simulink model "pd_path_sg"  (R2013b)
settings: Solver=ode45  StartTime=0.0  StopTime=10  RelTol=1e-3
undefined symbols (not defined in the file or in its folder): A, A2, B, C, D, EVAL, i, output_samp_bcoef, PCIN, reg_pk_lim, reg_plim, reg_scale, reg_sr_lim, reg_staclr, reg_txgain, THIS_DATE, W, X, Z
undefined symbols (not defined in the file): lut_address, lut_address_s5, reg_dltap
libraries: xbsIndex_r4 x3819, lut_ram_vhdl x32
(part 1 of 31)
settings Model: Creator=eyonfen  LastModifiedBy=Administrator
settings DataIOCC: SignalLoggingSaveFormat=ModelDataLogs
settings OptimizationCC: ExpressionDepthLimit=2147483647
settings DebuggingCC: FcnCallInpInsideContextMsg=EnableAllAsWarning  FrameProcessingCompatibilityMsg=error  StateNameClashWarn=warning
settings GRTTargetCC: CodeReplacementLibrary=None  CPPClassGenCompliant=on

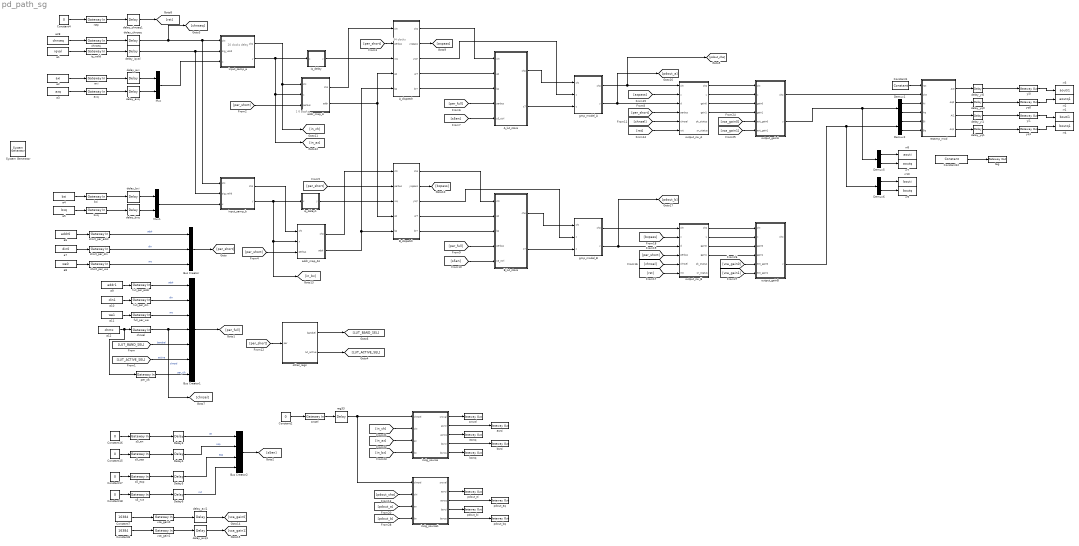
== system pd_path_sg ==
  note: 1 6 clocks
  note: 20 clocks delay
  note: 34 clocks
  " System Generator" : xbsIndex_r4/ System Generator  Tag=genX  xilinxfamily=zynquplus  part=xczu15eg  speed=-1LV-i-EVAL  package=ffvb1156  synthesis_tool=Vivado  clock_wrapper=Clock Enables  directory=../../../netlist/pd_path_sg  proj_type=Vivado  Synth_file=Vivado Synthesis Defaults  Impl_file=Vivado Implementation Defaults  testbench=off  simulink_period=1  sysclk_period=10  dcm_input_clock_period=10  incr_netlist=off  trim_vbits=Everywhere in SubSystem  dbl_ovrd=According to Block Masks  core_generation=According to Block Masks  run_coregen=off  deprecated_control=off  eval_field=0  block_type=sysgen
  A_dispatch : Subsystem  mask{para_band=0}
  A_lut_store : Subsystem  mask{band_sel=0}
  B_dispatch : Subsystem  mask{para_band=1}
  B_lut_store : Subsystem  mask{band_sel=1}
  Bus Creator : BusCreator  Inputs=3
  Bus Creator1 : BusCreator  Inputs=7
  Bus Creator2 : BusCreator
  Constant1 : xbsIndex_r4/Constant  const=0  gui_display_data_type=Boolean  arith_type=Boolean  n_bits=10  bin_pt=0  preci_type=Single  exp_width=8  frac_width=24  explicit_period=on  period=1  equ=P=C  opselect=C  inp2=PCIN>>17  opr=+  inp1=P  carry=CIN  dbl_ovrd=off  block_type=constant
  Constant12 : xbsIndex_r4/Constant  const=THIS_DATE  gui_display_data_type=Fixed-point  arith_type=Unsigned  n_bits=32  bin_pt=0  preci_type=Single  exp_width=8  frac_width=24  explicit_period=off  period=1  equ=P=C  opselect=C  inp2=PCIN>>17  opr=+  inp1=P  carry=CIN  dbl_ovrd=off  block_type=constant
  Constant{2,4,15..18} (6 alike) : Constant  Value=0
  Constant7 : Constant  Value=16384
  Constant8 : Constant  Value=16384
  Delay{3..6} (4 alike) : xbsIndex_r4/Delay  rst=off  infoeditControl=Selection of Reset will increase slice count due to use of real FFs and instead of SRLs  en=off  latency=1  reg_retiming=off  dbl_ovrd=off  block_type=delay
  Demux{1..2,5..6} (4 alike) : Demux  Outputs=2
  Mux : Mux  Inputs=2
  Mux1 : Mux  Inputs=2
  a1 : FromWorkspace  VariableName=iqval  Interpolate=off  OutputAfterFinalValue=Cyclic repetition
  a10 : FromWorkspace  VariableName=din1  Interpolate=off  OutputAfterFinalValue=Setting to zero
  a11 : FromWorkspace  VariableName=we1  Interpolate=off  OutputAfterFinalValue=Setting to zero
  a12 : FromWorkspace  VariableName=chntx  Interpolate=off  OutputAfterFinalValue=Cyclic repetition
  a2 : FromWorkspace  VariableName=axi  Interpolate=off  OutputAfterFinalValue=Setting to zero
  a28 : FromWorkspace  VariableName=chnseq  Interpolate=off  OutputAfterFinalValue=Cyclic repetition
  a3 : FromWorkspace  VariableName=axq  Interpolate=off  OutputAfterFinalValue=Setting to zero
  a4 : FromWorkspace  VariableName=bxi  Interpolate=off  OutputAfterFinalValue=Setting to zero
  a5 : FromWorkspace  VariableName=bxq  Interpolate=off  OutputAfterFinalValue=Setting to zero
  a6 : FromWorkspace  VariableName=addr0  Interpolate=off  OutputAfterFinalValue=Setting to zero
  a7 : FromWorkspace  VariableName=din0  Interpolate=off  OutputAfterFinalValue=Setting to zero
  a8 : FromWorkspace  VariableName=we0  Interpolate=off  OutputAfterFinalValue=Setting to zero
  a9 : FromWorkspace  VariableName=addr1  Interpolate=off  OutputAfterFinalValue=Setting to zero
  addr_map_A : Subsystem  mask{para_band=0}
  addr_map_A1 : Subsystem  mask{para_band=1}
  asrci : xbsIndex_r4/Gateway Out  inherit_from_input=off  hdl_port=on  rows=1  columns=1  UseAsDAC=off  DACChannel='1'  interface=None  automatic_assignment=on  address_offset=hex2dec('00')  intf_name=''  intf_description=''  timing_constraint=None  locs_specified=off  LOCs={}  io_standard={}  block_type=gatewayout
  asrcq : xbsIndex_r4/Gateway Out  inherit_from_input=off  hdl_port=on  rows=1  columns=1  UseAsDAC=off  DACChannel='1'  interface=None  automatic_assignment=on  address_offset=hex2dec('00')  intf_name=''  intf_description=''  timing_constraint=None  locs_specified=off  LOCs={}  io_standard={}  block_type=gatewayout
  axi : xbsIndex_r4/Gateway In  gui_display_data_type=Fixed-point  arith_type="Signed  (2's comp)"  n_bits=16  bin_pt=0  preci_type=Single  exp_width=8  frac_width=24  rows=1  columns=1  quantization="Round  (unbiased: +/- Inf)"  overflow=Saturate  period=1  UseAsADC=off  ADCChannel='1'  interface=None  automatic_assignment=on  address_offset=hex2dec('00')  intf_name=''  intf_description=''  default_value=0  timing_constraint=None  locs_specified=off  LOCs={}  io_standard={}  inherit_from_input=off  hdl_port=on  dbl_ovrd=off  block_type=gatewayin
  axq : xbsIndex_r4/Gateway In  gui_display_data_type=Fixed-point  arith_type="Signed  (2's comp)"  n_bits=16  bin_pt=0  preci_type=Single  exp_width=8  frac_width=24  rows=1  columns=1  quantization="Round  (unbiased: +/- Inf)"  overflow=Saturate  period=1  UseAsADC=off  ADCChannel='1'  interface=None  automatic_assignment=on  address_offset=hex2dec('00')  intf_name=''  intf_description=''  default_value=0  timing_constraint=None  locs_specified=off  LOCs={}  io_standard={}  inherit_from_input=off  hdl_port=on  dbl_ovrd=off  block_type=gatewayin
  bsrci : xbsIndex_r4/Gateway Out  inherit_from_input=off  hdl_port=on  rows=1  columns=1  UseAsDAC=off  DACChannel='1'  interface=None  automatic_assignment=on  address_offset=hex2dec('00')  intf_name=''  intf_description=''  timing_constraint=None  locs_specified=off  LOCs={}  io_standard={}  block_type=gatewayout
  bsrcq : xbsIndex_r4/Gateway Out  inherit_from_input=off  hdl_port=on  rows=1  columns=1  UseAsDAC=off  DACChannel='1'  interface=None  automatic_assignment=on  address_offset=hex2dec('00')  intf_name=''  intf_description=''  timing_constraint=None  locs_specified=off  LOCs={}  io_standard={}  block_type=gatewayout
  bxi : xbsIndex_r4/Gateway In  gui_display_data_type=Fixed-point  arith_type="Signed  (2's comp)"  n_bits=16  bin_pt=0  preci_type=Single  exp_width=8  frac_width=24  rows=1  columns=1  quantization="Round  (unbiased: +/- Inf)"  overflow=Saturate  period=1  UseAsADC=off  ADCChannel='1'  interface=None  automatic_assignment=on  address_offset=hex2dec('00')  intf_name=''  intf_description=''  default_value=0  timing_constraint=None  locs_specified=off  LOCs={}  io_standard={}  inherit_from_input=off  hdl_port=on  dbl_ovrd=off  block_type=gatewayin
  bxq : xbsIndex_r4/Gateway In  gui_display_data_type=Fixed-point  arith_type="Signed  (2's comp)"  n_bits=16  bin_pt=0  preci_type=Single  exp_width=8  frac_width=24  rows=1  columns=1  quantization="Round  (unbiased: +/- Inf)"  overflow=Saturate  period=1  UseAsADC=off  ADCChannel='1'  interface=None  automatic_assignment=on  address_offset=hex2dec('00')  intf_name=''  intf_description=''  default_value=0  timing_constraint=None  locs_specified=off  LOCs={}  io_standard={}  inherit_from_input=off  hdl_port=on  dbl_ovrd=off  block_type=gatewayin
  chnsel : xbsIndex_r4/Gateway In  gui_display_data_type=Fixed-point  arith_type=Unsigned  n_bits=1  bin_pt=0  preci_type=Single  exp_width=8  frac_width=24  rows=1  columns=1  quantization="Round  (unbiased: +/- Inf)"  overflow=Saturate  period=1  UseAsADC=off  ADCChannel='1'  interface=None  automatic_assignment=on  address_offset=hex2dec('00')  intf_name=''  intf_description=''  default_value=0  timing_constraint=None  locs_specified=off  LOCs={}  io_standard={}  inherit_from_input=off  hdl_port=on  dbl_ovrd=off  block_type=gatewayin
  chnseq : xbsIndex_r4/Gateway In  gui_display_data_type=Fixed-point  arith_type=Unsigned  n_bits=1  bin_pt=0  preci_type=Single  exp_width=8  frac_width=24  rows=1  columns=1  quantization="Round  (unbiased: +/- Inf)"  overflow=Saturate  period=1  UseAsADC=off  ADCChannel='1'  interface=None  automatic_assignment=on  address_offset=hex2dec('00')  intf_name=''  intf_description=''  default_value=0  timing_constraint=None  locs_specified=off  LOCs={}  io_standard={}  inherit_from_input=off  hdl_port=on  dbl_ovrd=off  block_type=gatewayin
  delay_axi : xbsIndex_r4/Delay  rst=off  infoeditControl=Selection of Reset will increase slice count due to use of real FFs and instead of SRLs  en=off  latency=1  reg_retiming=off  dbl_ovrd=off  block_type=delay
  delay_axi1 : xbsIndex_r4/Delay  rst=off  infoeditControl=Selection of Reset will increase slice count due to use of real FFs and instead of SRLs  en=off  latency=1  reg_retiming=off  dbl_ovrd=off  block_type=delay
  delay_axq : xbsIndex_r4/Delay  rst=off  infoeditControl=Selection of Reset will increase slice count due to use of real FFs and instead of SRLs  en=off  latency=1  reg_retiming=off  dbl_ovrd=off  block_type=delay
  delay_axq1 : xbsIndex_r4/Delay  rst=off  infoeditControl=Selection of Reset will increase slice count due to use of real FFs and instead of SRLs  en=off  latency=1  reg_retiming=off  dbl_ovrd=off  block_type=delay
  delay_bxi : xbsIndex_r4/Delay  rst=off  infoeditControl=Selection of Reset will increase slice count due to use of real FFs and instead of SRLs  en=off  latency=1  reg_retiming=off  dbl_ovrd=off  block_type=delay
  delay_bxq : xbsIndex_r4/Delay  rst=off  infoeditControl=Selection of Reset will increase slice count due to use of real FFs and instead of SRLs  en=off  latency=1  reg_retiming=off  dbl_ovrd=off  block_type=delay
  delay_chnseq : xbsIndex_r4/Delay  rst=off  infoeditControl=Selection of Reset will increase slice count due to use of real FFs and instead of SRLs  en=off  latency=1  reg_retiming=off  dbl_ovrd=off  block_type=delay
  delay_chnseq1 : xbsIndex_r4/Delay  rst=off  infoeditControl=Selection of Reset will increase slice count due to use of real FFs and instead of SRLs  en=off  latency=2  reg_retiming=off  dbl_ovrd=off  block_type=delay
      settings: infoedit=Hardware notes: A delay line is a chain, each link of which is an SRL16 or SRL32 followed by a flip-flop.
  delay_iqval : xbsIndex_r4/Delay  rst=off  infoeditControl=Selection of Reset will increase slice count due to use of real FFs and instead of SRLs  en=off  latency=1  reg_retiming=off  dbl_ovrd=off  block_type=delay
  delay_yi0 : xbsIndex_r4/Delay  rst=off  infoeditControl=Selection of Reset will increase slice count due to use of real FFs and instead of SRLs  en=off  latency=1  reg_retiming=off  dbl_ovrd=off  block_type=delay
  delay_yi1 : xbsIndex_r4/Delay  rst=off  infoeditControl=Selection of Reset will increase slice count due to use of real FFs and instead of SRLs  en=off  latency=1  reg_retiming=off  dbl_ovrd=off  block_type=delay
  delay_yq0 : xbsIndex_r4/Delay  rst=off  infoeditControl=Selection of Reset will increase slice count due to use of real FFs and instead of SRLs  en=off  latency=1  reg_retiming=off  dbl_ovrd=off  block_type=delay
  delay_yq1 : xbsIndex_r4/Delay  rst=off  infoeditControl=Selection of Reset will increase slice count due to use of real FFs and instead of SRLs  en=off  latency=1  reg_retiming=off  dbl_ovrd=off  block_type=delay
  full_per_addr : xbsIndex_r4/Gateway In  gui_display_data_type=Fixed-point  arith_type=Unsigned  n_bits=20  bin_pt=0  preci_type=Single  exp_width=8  frac_width=24  rows=1  columns=1  quantization="Round  (unbiased: +/- Inf)"  overflow=Saturate  period=1  UseAsADC=off  ADCChannel='1'  interface=None  automatic_assignment=on  address_offset=hex2dec('00')  intf_name=''  intf_description=''  default_value=0  timing_constraint=None  locs_specified=off  LOCs={}  io_standard={}  inherit_from_input=off  hdl_port=on  dbl_ovrd=off  block_type=gatewayin
  full_per_din : xbsIndex_r4/Gateway In  gui_display_data_type=Fixed-point  arith_type=Unsigned  n_bits=32  bin_pt=0  preci_type=Single  exp_width=8  frac_width=24  rows=1  columns=1  quantization="Round  (unbiased: +/- Inf)"  overflow=Saturate  period=1  UseAsADC=off  ADCChannel='1'  interface=None  automatic_assignment=on  address_offset=hex2dec('00')  intf_name=''  intf_description=''  default_value=0  timing_constraint=None  locs_specified=off  LOCs={}  io_standard={}  inherit_from_input=off  hdl_port=on  dbl_ovrd=off  block_type=gatewayin
  full_per_we : xbsIndex_r4/Gateway In  gui_display_data_type=Boolean  arith_type=Boolean  n_bits=1  bin_pt=0  preci_type=Single  exp_width=8  frac_width=24  rows=1  columns=1  quantization="Round  (unbiased: +/- Inf)"  overflow=Saturate  period=1  UseAsADC=off  ADCChannel='1'  interface=None  automatic_assignment=on  address_offset=hex2dec('00')  intf_name=''  intf_description=''  default_value=0  timing_constraint=None  locs_specified=off  LOCs={}  io_standard={}  inherit_from_input=off  hdl_port=on  dbl_ovrd=off  block_type=gatewayin
  gmp_model_A : Subsystem
  gmp_model_B : Subsystem
  input_samp_a : Subsystem
  input_samp_b : Subsystem
  insig_source : Subsystem
  insig_source1 : Subsystem
  iq_delay : Subsystem  mask{clocks=30}
  iq_delay1 : Subsystem  mask{clocks=30}
  iq_valid : xbsIndex_r4/Gateway In  gui_display_data_type=Fixed-point  arith_type=Unsigned  n_bits=1  bin_pt=0  preci_type=Single  exp_width=8  frac_width=24  rows=1  columns=1  quantization="Round  (unbiased: +/- Inf)"  overflow=Saturate  period=1  UseAsADC=off  ADCChannel='1'  interface=None  automatic_assignment=on  address_offset=hex2dec('00')  intf_name=''  intf_description=''  default_value=0  timing_constraint=None  locs_specified=off  LOCs={}  io_standard={}  inherit_from_input=off  hdl_port=on  dbl_ovrd=off  block_type=gatewayin
  other_regs : Subsystem
  output_gainA : Subsystem
  output_gainB : Subsystem
  output_sw_A : Subsystem  mask{para_band=0}
  output_sw_B : Subsystem  mask{para_band=1}
  pdout_ai : xbsIndex_r4/Gateway Out  inherit_from_input=off  hdl_port=on  rows=1  columns=1  UseAsDAC=off  DACChannel='1'  interface=None  automatic_assignment=on  address_offset=hex2dec('00')  intf_name=''  intf_description=''  timing_constraint=None  locs_specified=off  LOCs={}  io_standard={}  block_type=gatewayout
  pdout_aq : xbsIndex_r4/Gateway Out  inherit_from_input=off  hdl_port=on  rows=1  columns=1  UseAsDAC=off  DACChannel='1'  interface=None  automatic_assignment=on  address_offset=hex2dec('00')  intf_name=''  intf_description=''  timing_constraint=None  locs_specified=off  LOCs={}  io_standard={}  block_type=gatewayout
  pdout_bi : xbsIndex_r4/Gateway Out  inherit_from_input=off  hdl_port=on  rows=1  columns=1  UseAsDAC=off  DACChannel='1'  interface=None  automatic_assignment=on  address_offset=hex2dec('00')  intf_name=''  intf_description=''  timing_constraint=None  locs_specified=off  LOCs={}  io_standard={}  block_type=gatewayout
  pdout_bq : xbsIndex_r4/Gateway Out  inherit_from_input=off  hdl_port=on  rows=1  columns=1  UseAsDAC=off  DACChannel='1'  interface=None  automatic_assignment=on  address_offset=hex2dec('00')  intf_name=''  intf_description=''  timing_constraint=None  locs_specified=off  LOCs={}  io_standard={}  block_type=gatewayout
  per_clk : xbsIndex_r4/Gateway In  gui_display_data_type=Fixed-point  arith_type=Unsigned  n_bits=1  bin_pt=0  preci_type=Single  exp_width=8  frac_width=24  rows=1  columns=1  quantization="Round  (unbiased: +/- Inf)"  overflow=Saturate  period=1  UseAsADC=off  ADCChannel='1'  interface=None  automatic_assignment=on  address_offset=hex2dec('00')  intf_name=''  intf_description=''  default_value=0  timing_constraint=None  locs_specified=off  LOCs={}  io_standard={}  inherit_from_input=off  hdl_port=on  dbl_ovrd=off  block_type=gatewayin
  reg33 : xbsIndex_r4/Delay  rst=off  infoeditControl=Selection of Reset will increase slice count due to use of real FFs and instead of SRLs  en=off  latency=1  reg_retiming=off  dbl_ovrd=off  block_type=delay
  resamp_mod : Subsystem
  rr1 : ToWorkspace  VariableName=bouti1  SampleTime=-1
  rr10 : ToWorkspace  VariableName=bouti  SampleTime=-1
  rr2 : ToWorkspace  VariableName=aoutq1  SampleTime=-1
  rr3 : ToWorkspace  VariableName=aouti1  SampleTime=-1
  rr4 : ToWorkspace  VariableName=boutq1  SampleTime=-1
  rr7 : ToWorkspace  VariableName=aoutq  SampleTime=-1
  rr8 : ToWorkspace  VariableName=aouti  SampleTime=-1
  rr9 : ToWorkspace  VariableName=boutq  SampleTime=-1
  rstp : xbsIndex_r4/Gateway In  gui_display_data_type=Boolean  arith_type=Boolean  n_bits=1  bin_pt=0  preci_type=Single  exp_width=8  frac_width=24  rows=1  columns=1  quantization="Round  (unbiased: +/- Inf)"  overflow=Saturate  period=1  UseAsADC=off  ADCChannel='1'  interface=None  automatic_assignment=on  address_offset=hex2dec('00')  intf_name=''  intf_description=''  default_value=0  timing_constraint=None  locs_specified=off  LOCs={}  io_standard={}  inherit_from_input=off  hdl_port=on  dbl_ovrd=off  block_type=gatewayin
  s5_en : xbsIndex_r4/Gateway In  gui_display_data_type=Boolean  arith_type=Boolean  n_bits=1  bin_pt=0  preci_type=Single  exp_width=8  frac_width=24  rows=1  columns=1  quantization="Round  (unbiased: +/- Inf)"  overflow=Saturate  period=1  UseAsADC=off  ADCChannel='1'  interface=None  automatic_assignment=on  address_offset=hex2dec('00')  intf_name=''  intf_description=''  default_value=0  timing_constraint=None  locs_specified=off  LOCs={}  io_standard={}  inherit_from_input=off  hdl_port=on  dbl_ovrd=off  block_type=gatewayin
  s5_eop : xbsIndex_r4/Gateway In  gui_display_data_type=Boolean  arith_type=Boolean  n_bits=1  bin_pt=0  preci_type=Single  exp_width=8  frac_width=24  rows=1  columns=1  quantization="Round  (unbiased: +/- Inf)"  overflow=Saturate  period=1  UseAsADC=off  ADCChannel='1'  interface=None  automatic_assignment=on  address_offset=hex2dec('00')  intf_name=''  intf_description=''  default_value=0  timing_constraint=None  locs_specified=off  LOCs={}  io_standard={}  inherit_from_input=off  hdl_port=on  dbl_ovrd=off  block_type=gatewayin
  s5_nxt : xbsIndex_r4/Gateway In  gui_display_data_type=Boolean  arith_type=Boolean  n_bits=1  bin_pt=0  preci_type=Single  exp_width=8  frac_width=24  rows=1  columns=1  quantization="Round  (unbiased: +/- Inf)"  overflow=Saturate  period=1  UseAsADC=off  ADCChannel='1'  interface=None  automatic_assignment=on  address_offset=hex2dec('00')  intf_name=''  intf_description=''  default_value=0  timing_constraint=None  locs_specified=off  LOCs={}  io_standard={}  inherit_from_input=off  hdl_port=on  dbl_ovrd=off  block_type=gatewayin
  s5_sop : xbsIndex_r4/Gateway In  gui_display_data_type=Boolean  arith_type=Boolean  n_bits=1  bin_pt=0  preci_type=Single  exp_width=8  frac_width=24  rows=1  columns=1  quantization="Round  (unbiased: +/- Inf)"  overflow=Saturate  period=1  UseAsADC=off  ADCChannel='1'  interface=None  automatic_assignment=on  address_offset=hex2dec('00')  intf_name=''  intf_description=''  default_value=0  timing_constraint=None  locs_specified=off  LOCs={}  io_standard={}  inherit_from_input=off  hdl_port=on  dbl_ovrd=off  block_type=gatewayin
  short_per_addr : xbsIndex_r4/Gateway In  gui_display_data_type=Fixed-point  arith_type=Unsigned  n_bits=12  bin_pt=0  preci_type=Single  exp_width=8  frac_width=24  rows=1  columns=1  quantization="Round  (unbiased: +/- Inf)"  overflow=Saturate  period=1  UseAsADC=off  ADCChannel='1'  interface=None  automatic_assignment=on  address_offset=hex2dec('00')  intf_name=''  intf_description=''  default_value=0  timing_constraint=None  locs_specified=off  LOCs={}  io_standard={}  inherit_from_input=off  hdl_port=on  dbl_ovrd=off  block_type=gatewayin
  short_per_din : xbsIndex_r4/Gateway In  gui_display_data_type=Fixed-point  arith_type=Unsigned  n_bits=32  bin_pt=0  preci_type=Single  exp_width=8  frac_width=24  rows=1  columns=1  quantization="Round  (unbiased: +/- Inf)"  overflow=Saturate  period=1  UseAsADC=off  ADCChannel='1'  interface=None  automatic_assignment=on  address_offset=hex2dec('00')  intf_name=''  intf_description=''  default_value=0  timing_constraint=None  locs_specified=off  LOCs={}  io_standard={}  inherit_from_input=off  hdl_port=on  dbl_ovrd=off  block_type=gatewayin
  short_per_we : xbsIndex_r4/Gateway In  gui_display_data_type=Boolean  arith_type=Boolean  n_bits=1  bin_pt=0  preci_type=Single  exp_width=8  frac_width=24  rows=1  columns=1  quantization="Round  (unbiased: +/- Inf)"  overflow=Saturate  period=1  UseAsADC=off  ADCChannel='1'  interface=None  automatic_assignment=on  address_offset=hex2dec('00')  intf_name=''  intf_description=''  default_value=0  timing_constraint=None  locs_specified=off  LOCs={}  io_standard={}  inherit_from_input=off  hdl_port=on  dbl_ovrd=off  block_type=gatewayin
  srcsel : xbsIndex_r4/Gateway In  gui_display_data_type=Fixed-point  arith_type=Unsigned  n_bits=1  bin_pt=0  preci_type=Single  exp_width=8  frac_width=24  rows=1  columns=1  quantization="Round  (unbiased: +/- Inf)"  overflow=Saturate  period=1  UseAsADC=off  ADCChannel='1'  interface=None  automatic_assignment=on  address_offset=hex2dec('00')  intf_name=''  intf_description=''  default_value=0  timing_constraint=None  locs_specified=off  LOCs={}  io_standard={}  inherit_from_input=off  hdl_port=on  dbl_ovrd=off  block_type=gatewayin
  srcval : xbsIndex_r4/Gateway Out  inherit_from_input=off  hdl_port=on  rows=1  columns=1  UseAsDAC=off  DACChannel='1'  interface=None  automatic_assignment=on  address_offset=hex2dec('00')  intf_name=''  intf_description=''  timing_constraint=None  locs_specified=off  LOCs={}  io_standard={}  block_type=gatewayout
  tag : xbsIndex_r4/Gateway Out  inherit_from_input=off  hdl_port=on  rows=1  columns=1  UseAsDAC=off  DACChannel='1'  interface=None  automatic_assignment=on  address_offset=hex2dec('00')  intf_name=''  intf_description=''  timing_constraint=None  locs_specified=off  LOCs={}  io_standard={}  block_type=gatewayout
  vca_gain0 : xbsIndex_r4/Gateway In  gui_display_data_type=Fixed-point  arith_type=Unsigned  n_bits=16  bin_pt=0  preci_type=Single  exp_width=8  frac_width=24  rows=1  columns=1  quantization="Round  (unbiased: +/- Inf)"  overflow=Saturate  period=1  UseAsADC=off  ADCChannel='1'  interface=None  automatic_assignment=on  address_offset=hex2dec('00')  intf_name=''  intf_description=''  default_value=0  timing_constraint=None  locs_specified=off  LOCs={}  io_standard={}  inherit_from_input=off  hdl_port=on  dbl_ovrd=off  block_type=gatewayin
  vca_gain1 : xbsIndex_r4/Gateway In  gui_display_data_type=Fixed-point  arith_type=Unsigned  n_bits=16  bin_pt=0  preci_type=Single  exp_width=8  frac_width=24  rows=1  columns=1  quantization="Round  (unbiased: +/- Inf)"  overflow=Saturate  period=1  UseAsADC=off  ADCChannel='1'  interface=None  automatic_assignment=on  address_offset=hex2dec('00')  intf_name=''  intf_description=''  default_value=0  timing_constraint=None  locs_specified=off  LOCs={}  io_standard={}  inherit_from_input=off  hdl_port=on  dbl_ovrd=off  block_type=gatewayin
  yi0 : xbsIndex_r4/Gateway Out  inherit_from_input=off  hdl_port=on  rows=1  columns=1  UseAsDAC=off  DACChannel='1'  interface=None  automatic_assignment=on  address_offset=hex2dec('00')  intf_name=''  intf_description=''  timing_constraint=None  locs_specified=off  LOCs={}  io_standard={}  block_type=gatewayout
  yi1 : xbsIndex_r4/Gateway Out  inherit_from_input=off  hdl_port=on  rows=1  columns=1  UseAsDAC=off  DACChannel='1'  interface=None  automatic_assignment=on  address_offset=hex2dec('00')  intf_name=''  intf_description=''  timing_constraint=None  locs_specified=off  LOCs={}  io_standard={}  block_type=gatewayout
  yq0 : xbsIndex_r4/Gateway Out  inherit_from_input=off  hdl_port=on  rows=1  columns=1  UseAsDAC=off  DACChannel='1'  interface=None  automatic_assignment=on  address_offset=hex2dec('00')  intf_name=''  intf_description=''  timing_constraint=None  locs_specified=off  LOCs={}  io_standard={}  block_type=gatewayout
  yq1 : xbsIndex_r4/Gateway Out  inherit_from_input=off  hdl_port=on  rows=1  columns=1  UseAsDAC=off  DACChannel='1'  interface=None  automatic_assignment=on  address_offset=hex2dec('00')  intf_name=''  intf_description=''  timing_constraint=None  locs_specified=off  LOCs={}  io_standard={}  block_type=gatewayout
  wires:
  a7/1 -> short_per_din/1
  Constant12/1 -> tag/1
  a3/1 -> axq/1
  a2/1 -> axi/1
  axi/1 -> delay_axi/1
  axq/1 -> delay_axq/1
  a5/1 -> bxq/1
  a4/1 -> bxi/1
  bxi/1 -> delay_bxi/1
  bxq/1 -> delay_bxq/1
  a6/1 -> short_per_addr/1
  a8/1 -> short_per_we/1
  short_per_addr/1 -> Bus Creator/1  "addr"
  short_per_we/1 -> Bus Creator/3  "we"
  a10/1 -> full_per_din/1
  a9/1 -> full_per_addr/1
  a11/1 -> full_per_we/1
  full_per_addr/1 -> Bus Creator1/1  "addr"
  full_per_din/1 -> Bus Creator1/2  "din"
  full_per_we/1 -> Bus Creator1/3  "we"
  a1/1 -> iq_valid/1
  Mux/1 -> input_samp_a/3(x)
  Mux1/1 -> input_samp_b/3(x)
  iq_valid/1 -> delay_iqval/1
  input_samp_a/2(y) -> [in_ax], addr_map_A/2(x), iq_delay/1(x)
  a12/1 -> per_clk/1, chnsel/1
  chnsel/1 -> [chnsel], Bus Creator1/4  "chnsel"
  a28/1 -> chnseq/1
  [LUT_BAND_SEL] -> Bus Creator1/5  "bandsel"
  [LUT_ACTIVE_SEL] -> Bus Creator1/6  "active"
  input_samp_b/2(y) -> iq_delay1/1(x), addr_map_A1/2(x), [in_bx]
  Bus Creator/1 -> [per_short]
  Bus Creator1/1 -> [per_full]
  [per_short] -> addr_map_A/3(perbus)
  [per_short] -> A_dispatch/2(perbus)
  [per_short] -> addr_map_A1/3(perbus)
  [per_short] -> B_dispatch/2(perbus)
  Constant15/1 -> s5_sop/1
  s5_sop/1 -> Delay4/1
  Constant16/1 -> s5_en/1
  Constant17/1 -> s5_eop/1
  Constant18/1 -> s5_nxt/1
  s5_en/1 -> Delay3/1
  s5_nxt/1 -> Delay6/1
  s5_eop/1 -> Delay5/1
  Delay3/1 -> Bus Creator2/1  "en"
  Delay4/1 -> Bus Creator2/2  "sop"
  Delay5/1 -> Bus Creator2/3  "eop"
  Delay6/1 -> Bus Creator2/4  "nxt"
  Bus Creator2/1 -> [s5en]
  A_dispatch/4(ar7) -> A_lut_store/2(ap)
  A_dispatch/5(br7) -> A_lut_store/3(bp)
  chnseq/1 -> delay_chnseq/1
  [per_full] -> A_lut_store/4(perbus)
  [s5en] -> A_lut_store/5(s5_ctrl)
  B_dispatch/4(ar7) -> B_lut_store/2(ap)
  B_dispatch/5(br7) -> B_lut_store/3(bp)
  [per_full] -> B_lut_store/4(perbus)
  [s5en] -> B_lut_store/5(s5_ctrl)
  other_regs/2(lut_active) -> [LUT_ACTIVE_SEL]
  A_dispatch/1(cho) -> A_lut_store/1(chi)
  B_lut_store/2(c7) -> gmp_model_B/3(c)
  addr_map_A1/2(addr) -> B_dispatch/5(bp), A_dispatch/5(bp)
  [per_short] -> other_regs/1(per)
  iq_delay/1(y) -> A_dispatch/3(xiq)
  iq_delay1/1(y) -> B_dispatch/3(xiq)
  A_dispatch/3(yiq7) -> gmp_model_A/2(x)
  B_dispatch/3(yiq7) -> gmp_model_B/2(x)
  other_regs/1(bandsel) -> [LUT_BAND_SEL]
  per_clk/1 -> Bus Creator1/7  "per_clk"
  delay_axi/1 -> Mux/1
  delay_axq/1 -> Mux/2
  delay_bxi/1 -> Mux1/1
  delay_bxq/1 -> Mux1/2
  delay_iqval/1 -> input_samp_b/2(sig_valid), input_samp_a/2(sig_valid)
  delay_chnseq/1 -> [chnseq], input_samp_b/1(chi), input_samp_a/1(chi)
  short_per_din/1 -> Bus Creator/2  "din"
  Constant1/1 -> resamp_mod/1(rst)
  Demux1/1 -> resamp_mod/3(Ai)
  Demux1/2 -> resamp_mod/4(Aq)
  Demux2/1 -> resamp_mod/5(Bi)
  Demux2/2 -> resamp_mod/6(Bq)
  resamp_mod/1(Ai0) -> delay_yi0/1
  resamp_mod/2(Aq0) -> delay_yq0/1
  resamp_mod/3(Ai1) -> delay_yi1/1
  resamp_mod/4(Aq1) -> delay_yq1/1
  delay_yi0/1 -> yi0/1
  delay_yq0/1 -> yq0/1
  delay_yi1/1 -> yi1/1
  delay_yq1/1 -> yq1/1
  input_samp_a/1(cho) -> [in_ch], addr_map_A/1(chi)
  addr_map_A/1(cho) -> A_dispatch/1(chi)
  A_lut_store/1(cho) -> gmp_model_A/1(chi)
  A_lut_store/2(c7) -> gmp_model_A/3(c)
  addr_map_A/2(addr) -> B_dispatch/4(ap), A_dispatch/4(ap)
  input_samp_b/1(cho) -> addr_map_A1/1(chi)
  addr_map_A1/1(cho) -> B_dispatch/1(chi)
  B_dispatch/1(cho) -> B_lut_store/1(chi)
  B_lut_store/1(cho) -> gmp_model_B/1(chi)
  output_sw_A/1(cho) -> output_gainA/1(chi)
  output_sw_A/2(y) -> output_gainA/2(x)
  [vca_gain0] -> output_gainA/5(ext_gain0)
  [vca_gain1] -> output_gainA/6(ext_gain1)
  output_sw_A/3(gain0) -> output_gainA/3(gain0)
  output_sw_A/4(gain1) -> output_gainA/4(gain1)
  gmp_model_A/2(y) -> [pdout_a], output_sw_A/3(d)
  gmp_model_A/1(cho) -> [pdout_cha], output_sw_A/1(chi)
  output_gainA/2(y) -> Demux5/1, Demux1/1
  [per_short] -> output_sw_A/4(perbus)
  [chnsel] -> output_sw_A/5(chnsel)
  Constant4/1 -> rstp/1
  rstp/1 -> delay_chnseq1/1
  delay_chnseq1/1 -> [rst]
  [rst] -> output_sw_A/6(rst)
  A_dispatch/2(yiqpass) -> [axpass]
  [axpass] -> output_sw_A/2(x)
  B_dispatch/2(yiqpass) -> [bxpass]
  output_sw_B/1(cho) -> output_gainB/1(chi)
  output_sw_B/2(y) -> output_gainB/2(x)
  [vca_gain0] -> output_gainB/5(ext_gain0)
  [vca_gain1] -> output_gainB/6(ext_gain1)
  output_sw_B/3(gain0) -> output_gainB/3(gain0)
  output_sw_B/4(gain1) -> output_gainB/4(gain1)
  gmp_model_B/2(y) -> [pdout_b], output_sw_B/3(d)
  gmp_model_B/1(cho) -> output_sw_B/1(chi)
  [per_short] -> output_sw_B/4(perbus)
  [chnsel] -> output_sw_B/5(chnsel)
  [rst] -> output_sw_B/6(rst)
  [bxpass] -> output_sw_B/2(x)
  output_gainB/2(y) -> Demux6/1, Demux2/1
  reg33/1 -> insig_source1/1(chnsel), insig_source/1(chnsel)
  [in_ch] -> insig_source/2(chi)
  [in_ax] -> insig_source/3(ax)
  [in_bx] -> insig_source/4(bx)
  insig_source/1(srcval) -> srcval/1
  insig_source/2(asrci) -> asrci/1
  insig_source/3(asrcq) -> asrcq/1
  insig_source/4(bsrci) -> bsrci/1
  insig_source/5(bsrcq) -> bsrcq/1
  vca_gain0/1 -> delay_axi1/1
  vca_gain1/1 -> delay_axq1/1
  Constant7/1 -> vca_gain0/1
  Constant8/1 -> vca_gain1/1
  delay_axi1/1 -> [vca_gain0]
  delay_axq1/1 -> [vca_gain1]
  Demux5/1 -> rr8/1
  Demux5/2 -> rr7/1
  Demux6/1 -> rr10/1
  Demux6/2 -> rr9/1
  output_gainA/1(cho) -> resamp_mod/2(chn)
  yi0/1 -> rr3/1
  yq0/1 -> rr2/1
  yi1/1 -> rr1/1
  yq1/1 -> rr4/1
  srcsel/1 -> reg33/1
  Constant2/1 -> srcsel/1
  [pdout_cha] -> insig_source1/2(chi)
  [pdout_a] -> insig_source1/3(ax)
  [pdout_b] -> insig_source1/4(bx)
  insig_source1/2(asrci) -> pdout_ai/1
  insig_source1/3(asrcq) -> pdout_aq/1
  insig_source1/4(bsrci) -> pdout_bi/1
  insig_source1/5(bsrcq) -> pdout_bq/1

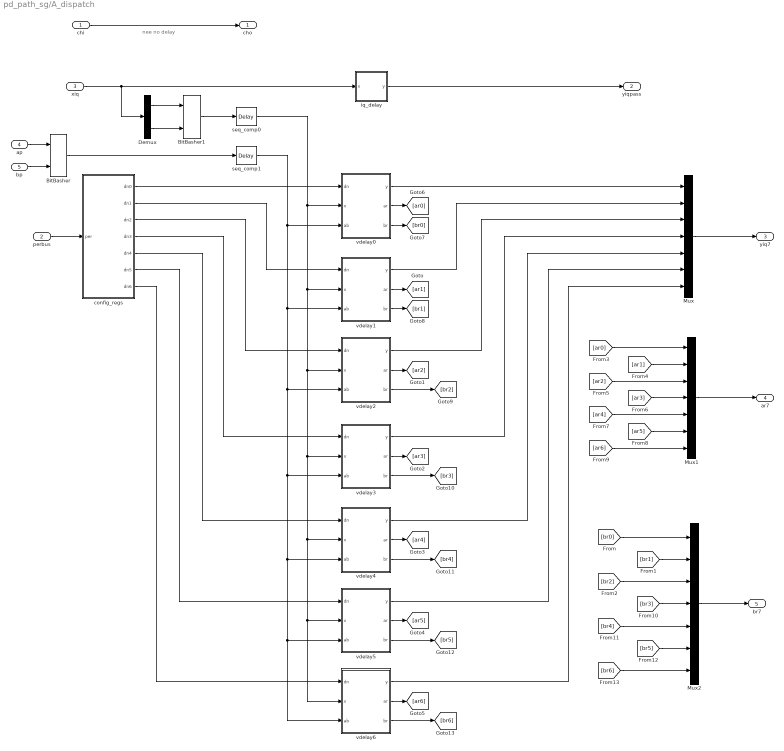
== system pd_path_sg/A_dispatch ==
  note: nee no delay
  chi : Inport
  perbus : Inport  Port=2
  xiq : Inport  Port=3
  ap : Inport  Port=4
  bp : Inport  Port=5
  BitBasher : xbsIndex_r4/BitBasher  bitexpr=a={b,c}  display_expr=off  sr_1=a  arith_type1=Unsigned  bin_pt1=0  sr_2=2  arith_type2=Unsigned  bin_pt2=0  sr_3=3  arith_type3=Unsigned  bin_pt3=0  sr_4=4  arith_type4=Unsigned  bin_pt4=0  dbl_ovrd=off  block_type=bitbasher
  BitBasher1 : xbsIndex_r4/BitBasher  bitexpr=a={b,c}  display_expr=off  sr_1=a  arith_type1=Unsigned  bin_pt1=0  sr_2=2  arith_type2=Unsigned  bin_pt2=0  sr_3=3  arith_type3=Unsigned  bin_pt3=0  sr_4=4  arith_type4=Unsigned  bin_pt4=0  dbl_ovrd=off  block_type=bitbasher
  Demux : Demux  Outputs=2
  Mux : Mux  Inputs=7
  Mux1 : Mux  Inputs=7
  Mux2 : Mux  Inputs=7
  config_regs : Subsystem
  iq_delay : Subsystem  mask{clocks=51}
  seq_comp0 : xbsIndex_r4/Delay  rst=off  infoeditControl=Selection of Reset will increase slice count due to use of real FFs and instead of SRLs  en=off  latency=1  reg_retiming=off  dbl_ovrd=off  block_type=delay
      settings: infoedit=Hardware notes: A delay line is a chain, each link of which is an SRL16 or SRL32 followed by a flip-flop.
  seq_comp1 : xbsIndex_r4/Delay  rst=off  infoeditControl=Selection of Reset will increase slice count due to use of real FFs and instead of SRLs  en=off  latency=1  reg_retiming=off  dbl_ovrd=off  block_type=delay
      settings: infoedit=Hardware notes: A delay line is a chain, each link of which is an SRL16 or SRL32 followed by a flip-flop.
  vdelay0 : Subsystem
  vdelay1 : Subsystem
  vdelay2 : Subsystem
  vdelay3 : Subsystem
  vdelay4 : Subsystem
  vdelay5 : Subsystem
  vdelay6 : Subsystem
  cho : Outport
  yiqpass : Outport  Port=2
  yiq7 : Outport  Port=3
  ar7 : Outport  Port=4
  br7 : Outport  Port=5
  wires:
  BitBasher1/1 -> seq_comp0/1
  Demux/1 -> BitBasher1/1
  Demux/2 -> BitBasher1/2
  [br6] -> Mux2/7
  [br5] -> Mux2/6
  [br3] -> Mux2/4
  [br4] -> Mux2/5
  vdelay6/3(br) -> [br6]
  vdelay5/3(br) -> [br5]
  vdelay4/3(br) -> [br4]
  vdelay3/3(br) -> [br3]
  vdelay2/3(br) -> [br2]
  vdelay1/3(br) -> [br1]
  vdelay6/2(ar) -> [ar6]
  vdelay5/2(ar) -> [ar5]
  vdelay4/2(ar) -> [ar4]
  [ar6] -> Mux1/7
  [ar5] -> Mux1/6
  [ar4] -> Mux1/5
  [ar3] -> Mux1/4
  [ar2] -> Mux1/3
  vdelay3/2(ar) -> [ar3]
  vdelay2/2(ar) -> [ar2]
  [ar1] -> Mux1/2
  vdelay1/2(ar) -> [ar1]
  [ar0] -> Mux1/1
  vdelay6/1(y) -> Mux/7
  vdelay5/1(y) -> Mux/6
  vdelay4/1(y) -> Mux/5
  config_regs/7(dn6) -> vdelay6/1(dn)
  config_regs/6(dn5) -> vdelay5/1(dn)
  config_regs/5(dn4) -> vdelay4/1(dn)
  config_regs/4(dn3) -> vdelay3/1(dn)
  config_regs/3(dn2) -> vdelay2/1(dn)
  config_regs/2(dn1) -> vdelay1/1(dn)
  [br2] -> Mux2/3
  [br1] -> Mux2/2
  [br0] -> Mux2/1
  Mux2/1 -> br7/1
  Mux1/1 -> ar7/1
  Mux/1 -> yiq7/1
  vdelay3/1(y) -> Mux/4
  vdelay2/1(y) -> Mux/3
  vdelay1/1(y) -> Mux/2
  vdelay0/1(y) -> Mux/1
  iq_delay/1(y) -> yiqpass/1
  config_regs/1(dn0) -> vdelay0/1(dn)
  BitBasher/1 -> seq_comp1/1
  bp/1 -> BitBasher/2
  ap/1 -> BitBasher/1
  xiq/1 -> iq_delay/1(x), Demux/1
  perbus/1 -> config_regs/1(per)
  seq_comp0/1 -> vdelay0/2(x), vdelay1/2(x), vdelay2/2(x), vdelay4/2(x), vdelay6/2(x), vdelay5/2(x), vdelay3/2(x)
  seq_comp1/1 -> vdelay0/3(ab), vdelay1/3(ab), vdelay2/3(ab), vdelay4/3(ab), vdelay6/3(ab), vdelay5/3(ab), vdelay3/3(ab)
  vdelay0/2(ar) -> [ar0]
  vdelay0/3(br) -> [br0]
  chi/1 -> cho/1

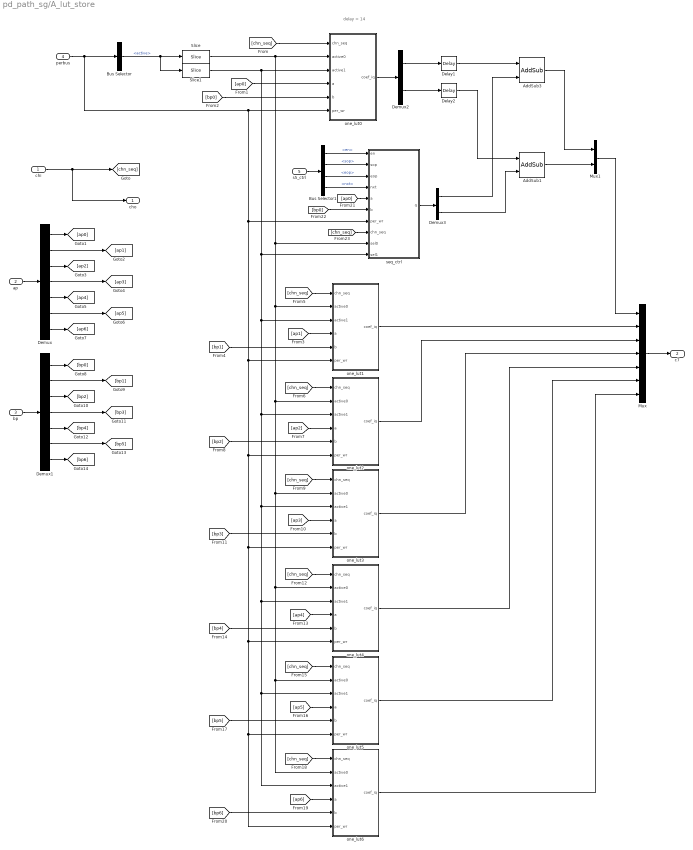
== system pd_path_sg/A_lut_store ==
  note: delay = 14
  chi : Inport
  ap : Inport  Port=2
  bp : Inport  Port=3
  perbus : Inport  Port=4
  s5_ctrl : Inport  Port=5
  AddSub1 : xbsIndex_r4/AddSub  mode=Addition  use_carryin=off  use_carryout=off  en=off  latency=1  precision=User Defined  arith_type="Signed  (2's comp)"  n_bits=16  bin_pt=0  quantization=Truncate  overflow=Wrap  use_behavioral_HDL=off  hw_selection=Fabric  pipelined=off  dbl_ovrd=off  block_type=addsub
  AddSub3 : xbsIndex_r4/AddSub  mode=Addition  use_carryin=off  use_carryout=off  en=off  latency=1  precision=User Defined  arith_type="Signed  (2's comp)"  n_bits=16  bin_pt=0  quantization=Truncate  overflow=Wrap  use_behavioral_HDL=off  hw_selection=Fabric  pipelined=off  dbl_ovrd=off  block_type=addsub
  Bus Selector : BusSelector  OutputSignals=active
  Bus Selector1 : BusSelector  OutputSignals=en,sop,eop,nxt
  Delay1 : xbsIndex_r4/Delay  rst=off  infoeditControl=Selection of Reset will increase slice count due to use of real FFs and instead of SRLs  en=off  latency=1  reg_retiming=off  dbl_ovrd=off  block_type=delay
  Delay2 : xbsIndex_r4/Delay  rst=off  infoeditControl=Selection of Reset will increase slice count due to use of real FFs and instead of SRLs  en=off  latency=1  reg_retiming=off  dbl_ovrd=off  block_type=delay
  Demux : Demux  Outputs=7
  Demux1 : Demux  Outputs=7
  Demux2 : Demux  Outputs=2
  Demux3 : Demux  Outputs=2
  Mux : Mux  Inputs=7
  Mux1 : Mux  Inputs=2
  Slice : xbsIndex_r4/Slice  nbits=1  boolean_output=off  mode=Lower Bit Location + Width  bit1=0  base1=MSB of Input  bit0=2*band_sel + 0  base0=LSB of Input  dbl_ovrd=off  block_type=slice
  Slice1 : xbsIndex_r4/Slice  nbits=1  boolean_output=off  mode=Lower Bit Location + Width  bit1=0  base1=MSB of Input  bit0=2*band_sel + 1  base0=LSB of Input  dbl_ovrd=off  block_type=slice
  one_lut0 : Subsystem  mask{lut_addr=lut_address(1)}
  one_lut1 : Subsystem  mask{lut_addr=lut_address(2)}
  one_lut2 : Subsystem  mask{lut_addr=lut_address(3)}
  one_lut3 : Subsystem  mask{lut_addr=lut_address(4)}
  one_lut4 : Subsystem  mask{lut_addr=lut_address(5)}
  one_lut5 : Subsystem  mask{lut_addr=lut_address(6)}
  one_lut6 : Subsystem  mask{lut_addr=lut_address(7)}
  seq_ctrl : Subsystem
  cho : Outport
  c7 : Outport  Port=2
  wires:
  ap/1 -> Demux/1
  bp/1 -> Demux1/1
  Mux/1 -> c7/1
  s5_ctrl/1 -> Bus Selector1/1
  Bus Selector1/1 -> seq_ctrl/1(en)  "<en>"
  Bus Selector1/2 -> seq_ctrl/2(sop)  "<sop>"
  Bus Selector1/3 -> seq_ctrl/3(eop)  "<eop>"
  Bus Selector1/4 -> seq_ctrl/4(nxt)  "<nxt>"
  perbus/1 -> Bus Selector/1, one_lut1/6(per_wr), one_lut2/6(per_wr), one_lut3/6(per_wr), one_lut4/6(per_wr), one_lut6/6(per_wr), one_lut5/6(per_wr), seq_ctrl/7(per_wr), one_lut0/6(per_wr)
  Bus Selector/1 -> Slice1/1, Slice/1  "<active>"
  chi/1 -> cho/1, [chn_seq]
  [chn_seq] -> one_lut0/1(chn_seq)
  Demux/1 -> [ap0]
  Demux/2 -> [ap1]
  Demux/3 -> [ap2]
  Demux/4 -> [ap3]
  Demux/5 -> [ap4]
  Demux/6 -> [ap5]
  Demux/7 -> [ap6]
  [ap0] -> one_lut0/4(a)
  [bp0] -> one_lut0/5(b)
  Demux1/2 -> [bp1]
  Demux1/4 -> [bp3]
  Demux1/6 -> [bp5]
  Demux1/1 -> [bp0]
  Demux1/3 -> [bp2]
  Demux1/5 -> [bp4]
  Demux1/7 -> [bp6]
  [ap1] -> one_lut1/4(a)
  [bp1] -> one_lut1/5(b)
  [chn_seq] -> one_lut1/1(chn_seq)
  [chn_seq] -> one_lut2/1(chn_seq)
  [ap2] -> one_lut2/4(a)
  [bp2] -> one_lut2/5(b)
  [chn_seq] -> one_lut3/1(chn_seq)
  [ap3] -> one_lut3/4(a)
  [bp3] -> one_lut3/5(b)
  [chn_seq] -> one_lut4/1(chn_seq)
  [ap4] -> one_lut4/4(a)
  [bp4] -> one_lut4/5(b)
  [chn_seq] -> one_lut5/1(chn_seq)
  [ap5] -> one_lut5/4(a)
  [bp5] -> one_lut5/5(b)
  [chn_seq] -> one_lut6/1(chn_seq)
  [ap6] -> one_lut6/4(a)
  [bp6] -> one_lut6/5(b)
  Mux1/1 -> Mux/1
  seq_ctrl/1(q) -> Demux3/1
  Demux3/1 -> AddSub3/2
  Demux3/2 -> AddSub1/2
  AddSub3/1 -> Mux1/1
  AddSub1/1 -> Mux1/2
  [ap0] -> seq_ctrl/5(a)
  [bp0] -> seq_ctrl/6(b)
  [chn_seq] -> seq_ctrl/8(chn_seq)
  one_lut0/1(coef_iq) -> Demux2/1
  Demux2/1 -> Delay1/1
  Demux2/2 -> Delay2/1
  one_lut2/1(coef_iq) -> Mux/3
  one_lut3/1(coef_iq) -> Mux/4
  one_lut4/1(coef_iq) -> Mux/5
  one_lut5/1(coef_iq) -> Mux/6
  one_lut6/1(coef_iq) -> Mux/7
  one_lut1/1(coef_iq) -> Mux/2
  Delay1/1 -> AddSub3/1
  Delay2/1 -> AddSub1/1
  Slice/1 -> one_lut0/2(active0), one_lut1/2(active0), one_lut2/2(active0), one_lut3/2(active0), one_lut4/2(active0), one_lut6/2(active0), one_lut5/2(active0), seq_ctrl/9(sel0)
  Slice1/1 -> one_lut0/3(active1), seq_ctrl/10(sel1), one_lut1/3(active1), one_lut2/3(active1), one_lut3/3(active1), one_lut4/3(active1), one_lut6/3(active1), one_lut5/3(active1)

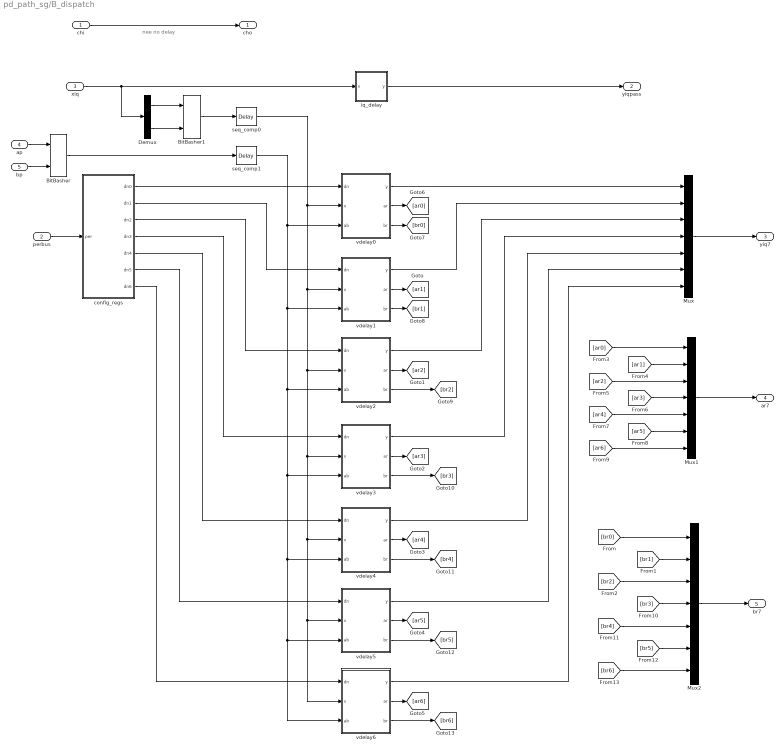
== system pd_path_sg/B_dispatch ==
  note: nee no delay
  chi : Inport
  perbus : Inport  Port=2
  xiq : Inport  Port=3
  ap : Inport  Port=4
  bp : Inport  Port=5
  BitBasher : xbsIndex_r4/BitBasher  bitexpr=a={b,c}  display_expr=off  sr_1=a  arith_type1=Unsigned  bin_pt1=0  sr_2=2  arith_type2=Unsigned  bin_pt2=0  sr_3=3  arith_type3=Unsigned  bin_pt3=0  sr_4=4  arith_type4=Unsigned  bin_pt4=0  dbl_ovrd=off  block_type=bitbasher
  BitBasher1 : xbsIndex_r4/BitBasher  bitexpr=a={b,c}  display_expr=off  sr_1=a  arith_type1=Unsigned  bin_pt1=0  sr_2=2  arith_type2=Unsigned  bin_pt2=0  sr_3=3  arith_type3=Unsigned  bin_pt3=0  sr_4=4  arith_type4=Unsigned  bin_pt4=0  dbl_ovrd=off  block_type=bitbasher
  Demux : Demux  Outputs=2
  Mux : Mux  Inputs=7
  Mux1 : Mux  Inputs=7
  Mux2 : Mux  Inputs=7
  config_regs : Subsystem
  iq_delay : Subsystem  mask{clocks=51}
  seq_comp0 : xbsIndex_r4/Delay  rst=off  infoeditControl=Selection of Reset will increase slice count due to use of real FFs and instead of SRLs  en=off  latency=1  reg_retiming=off  dbl_ovrd=off  block_type=delay
      settings: infoedit=Hardware notes: A delay line is a chain, each link of which is an SRL16 or SRL32 followed by a flip-flop.
  seq_comp1 : xbsIndex_r4/Delay  rst=off  infoeditControl=Selection of Reset will increase slice count due to use of real FFs and instead of SRLs  en=off  latency=1  reg_retiming=off  dbl_ovrd=off  block_type=delay
      settings: infoedit=Hardware notes: A delay line is a chain, each link of which is an SRL16 or SRL32 followed by a flip-flop.
  vdelay0 : Subsystem
  vdelay1 : Subsystem
  vdelay2 : Subsystem
  vdelay3 : Subsystem
  vdelay4 : Subsystem
  vdelay5 : Subsystem
  vdelay6 : Subsystem
  cho : Outport
  yiqpass : Outport  Port=2
  yiq7 : Outport  Port=3
  ar7 : Outport  Port=4
  br7 : Outport  Port=5
  wires:
  chi/1 -> cho/1
  vdelay0/3(br) -> [br0]
  vdelay0/2(ar) -> [ar0]
  seq_comp1/1 -> vdelay0/3(ab), vdelay1/3(ab), vdelay2/3(ab), vdelay3/3(ab), vdelay4/3(ab), vdelay6/3(ab), vdelay5/3(ab)
  seq_comp0/1 -> vdelay0/2(x), vdelay1/2(x), vdelay2/2(x), vdelay3/2(x), vdelay4/2(x), vdelay6/2(x), vdelay5/2(x)
  perbus/1 -> config_regs/1(per)
  xiq/1 -> Demux/1, iq_delay/1(x)
  ap/1 -> BitBasher/1
  bp/1 -> BitBasher/2
  BitBasher/1 -> seq_comp1/1
  config_regs/1(dn0) -> vdelay0/1(dn)
  iq_delay/1(y) -> yiqpass/1
  vdelay0/1(y) -> Mux/1
  vdelay1/1(y) -> Mux/2
  vdelay2/1(y) -> Mux/3
  vdelay3/1(y) -> Mux/4
  Mux/1 -> yiq7/1
  Mux1/1 -> ar7/1
  Mux2/1 -> br7/1
  [br0] -> Mux2/1
  [br1] -> Mux2/2
  [br2] -> Mux2/3
  config_regs/2(dn1) -> vdelay1/1(dn)
  config_regs/3(dn2) -> vdelay2/1(dn)
  config_regs/4(dn3) -> vdelay3/1(dn)
  config_regs/5(dn4) -> vdelay4/1(dn)
  config_regs/6(dn5) -> vdelay5/1(dn)
  config_regs/7(dn6) -> vdelay6/1(dn)
  vdelay4/1(y) -> Mux/5
  vdelay5/1(y) -> Mux/6
  vdelay6/1(y) -> Mux/7
  [ar0] -> Mux1/1
  vdelay1/2(ar) -> [ar1]
  [ar1] -> Mux1/2
  vdelay2/2(ar) -> [ar2]
  vdelay3/2(ar) -> [ar3]
  [ar2] -> Mux1/3
  [ar3] -> Mux1/4
  [ar4] -> Mux1/5
  [ar5] -> Mux1/6
  [ar6] -> Mux1/7
  vdelay4/2(ar) -> [ar4]
  vdelay5/2(ar) -> [ar5]
  vdelay6/2(ar) -> [ar6]
  vdelay1/3(br) -> [br1]
  vdelay2/3(br) -> [br2]
  vdelay3/3(br) -> [br3]
  vdelay4/3(br) -> [br4]
  vdelay5/3(br) -> [br5]
  vdelay6/3(br) -> [br6]
  [br4] -> Mux2/5
  [br3] -> Mux2/4
  [br5] -> Mux2/6
  [br6] -> Mux2/7
  Demux/2 -> BitBasher1/2
  Demux/1 -> BitBasher1/1
  BitBasher1/1 -> seq_comp0/1

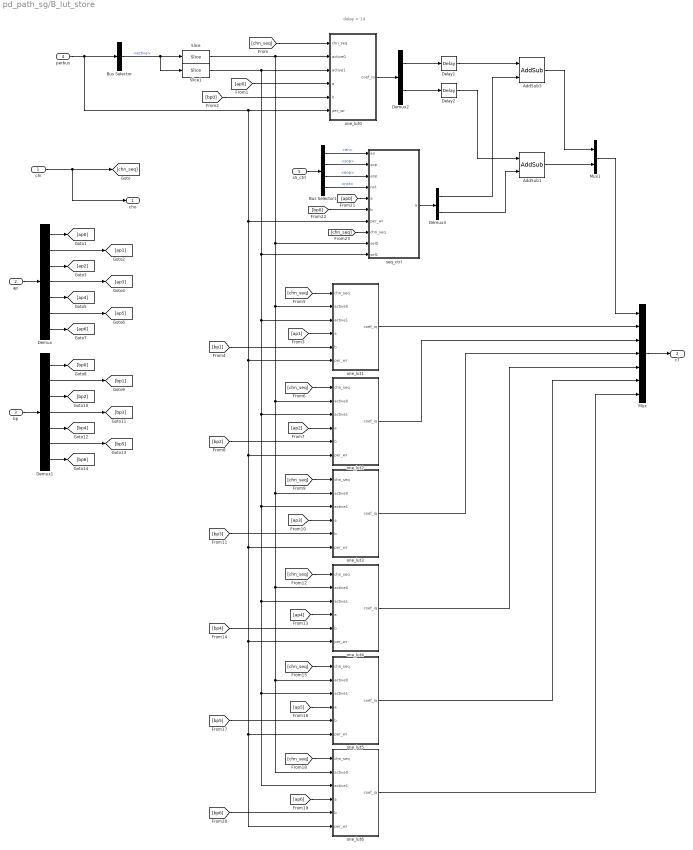
== system pd_path_sg/B_lut_store ==
  note: delay = 14
  chi : Inport
  ap : Inport  Port=2
  bp : Inport  Port=3
  perbus : Inport  Port=4
  s5_ctrl : Inport  Port=5
  AddSub1 : xbsIndex_r4/AddSub  mode=Addition  use_carryin=off  use_carryout=off  en=off  latency=1  precision=User Defined  arith_type="Signed  (2's comp)"  n_bits=16  bin_pt=0  quantization=Truncate  overflow=Wrap  use_behavioral_HDL=off  hw_selection=Fabric  pipelined=off  dbl_ovrd=off  block_type=addsub
  AddSub3 : xbsIndex_r4/AddSub  mode=Addition  use_carryin=off  use_carryout=off  en=off  latency=1  precision=User Defined  arith_type="Signed  (2's comp)"  n_bits=16  bin_pt=0  quantization=Truncate  overflow=Wrap  use_behavioral_HDL=off  hw_selection=Fabric  pipelined=off  dbl_ovrd=off  block_type=addsub
  Bus Selector : BusSelector  OutputSignals=active
  Bus Selector1 : BusSelector  OutputSignals=en,sop,eop,nxt
  Delay1 : xbsIndex_r4/Delay  rst=off  infoeditControl=Selection of Reset will increase slice count due to use of real FFs and instead of SRLs  en=off  latency=1  reg_retiming=off  dbl_ovrd=off  block_type=delay
  Delay2 : xbsIndex_r4/Delay  rst=off  infoeditControl=Selection of Reset will increase slice count due to use of real FFs and instead of SRLs  en=off  latency=1  reg_retiming=off  dbl_ovrd=off  block_type=delay
  Demux : Demux  Outputs=7
  Demux1 : Demux  Outputs=7
  Demux2 : Demux  Outputs=2
  Demux3 : Demux  Outputs=2
  Mux : Mux  Inputs=7
  Mux1 : Mux  Inputs=2
  Slice : xbsIndex_r4/Slice  nbits=1  boolean_output=off  mode=Lower Bit Location + Width  bit1=0  base1=MSB of Input  bit0=2*band_sel + 0  base0=LSB of Input  dbl_ovrd=off  block_type=slice
  Slice1 : xbsIndex_r4/Slice  nbits=1  boolean_output=off  mode=Lower Bit Location + Width  bit1=0  base1=MSB of Input  bit0=2*band_sel + 1  base0=LSB of Input  dbl_ovrd=off  block_type=slice
  one_lut0 : Subsystem  mask{lut_addr=lut_address(1)}
  one_lut1 : Subsystem  mask{lut_addr=lut_address(2)}
  one_lut2 : Subsystem  mask{lut_addr=lut_address(3)}
  one_lut3 : Subsystem  mask{lut_addr=lut_address(4)}
  one_lut4 : Subsystem  mask{lut_addr=lut_address(5)}
  one_lut5 : Subsystem  mask{lut_addr=lut_address(6)}
  one_lut6 : Subsystem  mask{lut_addr=lut_address(7)}
  seq_ctrl : Subsystem
  cho : Outport
  c7 : Outport  Port=2
  wires:
  Slice1/1 -> one_lut5/3(active1), one_lut6/3(active1), one_lut4/3(active1), one_lut3/3(active1), one_lut2/3(active1), one_lut1/3(active1), seq_ctrl/10(sel1), one_lut0/3(active1)
  Slice/1 -> seq_ctrl/9(sel0), one_lut5/2(active0), one_lut6/2(active0), one_lut4/2(active0), one_lut3/2(active0), one_lut2/2(active0), one_lut1/2(active0), one_lut0/2(active0)
  Delay2/1 -> AddSub1/1
  Delay1/1 -> AddSub3/1
  one_lut1/1(coef_iq) -> Mux/2
  one_lut6/1(coef_iq) -> Mux/7
  one_lut5/1(coef_iq) -> Mux/6
  one_lut4/1(coef_iq) -> Mux/5
  one_lut3/1(coef_iq) -> Mux/4
  one_lut2/1(coef_iq) -> Mux/3
  Demux2/2 -> Delay2/1
  Demux2/1 -> Delay1/1
  one_lut0/1(coef_iq) -> Demux2/1
  [chn_seq] -> seq_ctrl/8(chn_seq)
  [bp0] -> seq_ctrl/6(b)
  [ap0] -> seq_ctrl/5(a)
  AddSub1/1 -> Mux1/2
  AddSub3/1 -> Mux1/1
  Demux3/2 -> AddSub1/2
  Demux3/1 -> AddSub3/2
  seq_ctrl/1(q) -> Demux3/1
  Mux1/1 -> Mux/1
  [bp6] -> one_lut6/5(b)
  [ap6] -> one_lut6/4(a)
  [chn_seq] -> one_lut6/1(chn_seq)
  [bp5] -> one_lut5/5(b)
  [ap5] -> one_lut5/4(a)
  [chn_seq] -> one_lut5/1(chn_seq)
  [bp4] -> one_lut4/5(b)
  [ap4] -> one_lut4/4(a)
  [chn_seq] -> one_lut4/1(chn_seq)
  [bp3] -> one_lut3/5(b)
  [ap3] -> one_lut3/4(a)
  [chn_seq] -> one_lut3/1(chn_seq)
  [bp2] -> one_lut2/5(b)
  [ap2] -> one_lut2/4(a)
  [chn_seq] -> one_lut2/1(chn_seq)
  [chn_seq] -> one_lut1/1(chn_seq)
  [bp1] -> one_lut1/5(b)
  [ap1] -> one_lut1/4(a)
  Demux1/7 -> [bp6]
  Demux1/5 -> [bp4]
  Demux1/3 -> [bp2]
  Demux1/1 -> [bp0]
  Demux1/6 -> [bp5]
  Demux1/4 -> [bp3]
  Demux1/2 -> [bp1]
  [bp0] -> one_lut0/5(b)
  [ap0] -> one_lut0/4(a)
  Demux/7 -> [ap6]
  Demux/6 -> [ap5]
  Demux/5 -> [ap4]
  Demux/4 -> [ap3]
  Demux/3 -> [ap2]
  Demux/2 -> [ap1]
  Demux/1 -> [ap0]
  [chn_seq] -> one_lut0/1(chn_seq)
  chi/1 -> [chn_seq], cho/1
  Bus Selector/1 -> Slice/1, Slice1/1  "<active>"
  perbus/1 -> one_lut0/6(per_wr), seq_ctrl/7(per_wr), one_lut5/6(per_wr), one_lut6/6(per_wr), one_lut4/6(per_wr), one_lut3/6(per_wr), one_lut2/6(per_wr), one_lut1/6(per_wr), Bus Selector/1
  Bus Selector1/4 -> seq_ctrl/4(nxt)  "<nxt>"
  Bus Selector1/3 -> seq_ctrl/3(eop)  "<eop>"
  Bus Selector1/2 -> seq_ctrl/2(sop)  "<sop>"
  Bus Selector1/1 -> seq_ctrl/1(en)  "<en>"
  s5_ctrl/1 -> Bus Selector1/1
  Mux/1 -> c7/1
  bp/1 -> Demux1/1
  ap/1 -> Demux/1

== system pd_path_sg/addr_map_A ==
  note: need no delay
  note: 22bit
  chi : Inport
  x : Inport  Port=2
  perbus : Inport  Port=3
  Delay2 : xbsIndex_r4/Delay  rst=off  infoeditControl=Selection of Reset will increase slice count due to use of real FFs and instead of SRLs  en=off  latency=1  reg_retiming=off  dbl_ovrd=off  block_type=delay
  Delay3 : xbsIndex_r4/Delay  rst=off  infoeditControl=Selection of Reset will increase slice count due to use of real FFs and instead of SRLs  en=off  latency=1  reg_retiming=off  dbl_ovrd=off  block_type=delay
  Demux : Demux  Outputs=2
  Slice2 : xbsIndex_r4/Slice  nbits=10  boolean_output=off  mode=Lower Bit Location + Width  bit1=0  base1=MSB of Input  bit0=4  base0=LSB of Input  dbl_ovrd=off  block_type=slice
  config_regs : Subsystem
  gain_scaling : Subsystem
  mapping : Subsystem
  pwr : Subsystem
  saturation : Subsystem
  cho : Outport
  addr : Outport  Port=2
  wires:
  perbus/1 -> config_regs/1(per)
  saturation/1(q) -> mapping/1(d)
  gain_scaling/1(q) -> saturation/1(d)
  x/1 -> Demux/1
  Demux/1 -> pwr/1(xi)
  Demux/2 -> pwr/2(xq)
  pwr/1(q) -> Delay2/1
  config_regs/1(scale) -> gain_scaling/2(scale)
  Delay2/1 -> gain_scaling/1(d)
  mapping/1(q) -> Slice2/1
  Delay3/1 -> addr/1
  chi/1 -> cho/1
  Slice2/1 -> Delay3/1

== system pd_path_sg/addr_map_A1 ==
  note: 22bit
  note: need no delay
  chi : Inport
  x : Inport  Port=2
  perbus : Inport  Port=3
  Delay2 : xbsIndex_r4/Delay  rst=off  infoeditControl=Selection of Reset will increase slice count due to use of real FFs and instead of SRLs  en=off  latency=1  reg_retiming=off  dbl_ovrd=off  block_type=delay
  Delay3 : xbsIndex_r4/Delay  rst=off  infoeditControl=Selection of Reset will increase slice count due to use of real FFs and instead of SRLs  en=off  latency=1  reg_retiming=off  dbl_ovrd=off  block_type=delay
  Demux : Demux  Outputs=2
  Slice2 : xbsIndex_r4/Slice  nbits=10  boolean_output=off  mode=Lower Bit Location + Width  bit1=0  base1=MSB of Input  bit0=4  base0=LSB of Input  dbl_ovrd=off  block_type=slice
  config_regs : Subsystem
  gain_scaling : Subsystem
  mapping : Subsystem
  pwr : Subsystem
  saturation : Subsystem
  cho : Outport
  addr : Outport  Port=2
  wires:
  Slice2/1 -> Delay3/1
  chi/1 -> cho/1
  Delay3/1 -> addr/1
  mapping/1(q) -> Slice2/1
  Delay2/1 -> gain_scaling/1(d)
  config_regs/1(scale) -> gain_scaling/2(scale)
  pwr/1(q) -> Delay2/1
  Demux/2 -> pwr/2(xq)
  Demux/1 -> pwr/1(xi)
  x/1 -> Demux/1
  gain_scaling/1(q) -> saturation/1(d)
  saturation/1(q) -> mapping/1(d)
  perbus/1 -> config_regs/1(per)
